simulink model "pvinverter_det"  (R2014a)
settings: Solver=ode23tb  StartTime=0.0  StopTime=0.2  FixedStep=Ts  MaxStep=1e-3  RelTol=1e-4
PreLoadFcn:
  | PVArrayIsc = 5;
  | PVArrayVoc = 21.6;
  | PVArrayRs = 0.036;
  | Tcircuit = 27.15;
  | Toffset = -2;
  | TIPH1 = 0.001;
  | TXIS1 = 3;
  | TRS1 = 0;
  | Ts = 1e-6;
  | load('InvBusObject');
  | load('PVBusObject');
InitFcn:
  | Ts = 1e-6;
StartFcn:
  | tic;
StopFcn:
  | toc;
undefined symbols (not defined in the file or in its folder): sigbuilder_block
libraries: powerlib x13, powerlib_meascontrol x2
settings Model: Creator=cosorio  LastModifiedBy=cosorio
settings DataIOCC: LimitDataPoints=off  SignalLoggingSaveFormat=ModelDataLogs  SaveOutput=off  SignalLogging=off  SaveTime=off
settings OptimizationCC: ExpressionDepthLimit=2147483647
settings DebuggingCC: UnderspecifiedInitializationDetection=Classic  SolverPrmCheckMsg=none  FcnCallInpInsideContextMsg=UseLocalSettings  StateNameClashWarn=warning
settings GRTTargetCC: CombineOutputUpdateFcns=off  GRTInterface=on

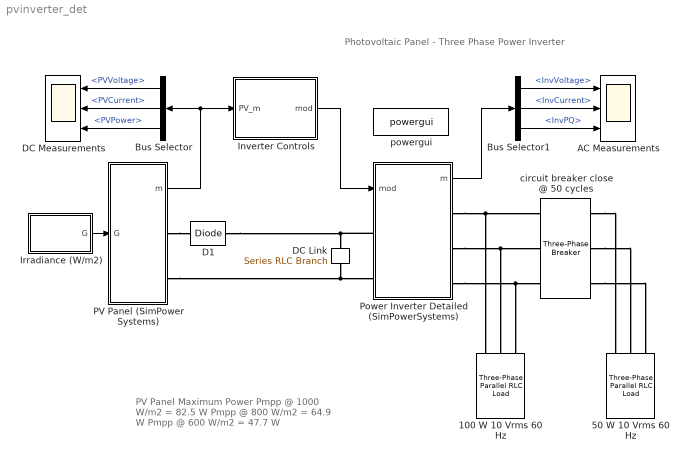
== system pvinverter_det ==
  note: Photovoltaic Panel - Three Phase Power Inverter
  note: PV Panel Maximum Power
      | Pmpp @ 1000 W/m2 = 82.5 W
      | Pmpp @ 800 W/m2 = 64.9 W
      | Pmpp @ 600 W/m2 = 47.7 W
  100 W 10 Vrms 60 Hz : powerlib/Elements/Three-Phase Parallel RLC Load  LConnTagsString=A|B|C  Configuration=Y (grounded)  NominalVoltage=10  NominalFrequency=60  ActivePower=100  InductivePower=0  CapacitivePower=0  Measurements=None  LoadType=constant Z
  50 W 10 Vrms 60 Hz : powerlib/Elements/Three-Phase Parallel RLC Load  LConnTagsString=A|B|C  Configuration=Y (grounded)  NominalVoltage=10  NominalFrequency=60  ActivePower=50  InductivePower=0  CapacitivePower=0  Measurements=None  LoadType=constant Z
  AC Measurements : Scope  NumInputPorts=3
      settings: YMin=-10~-10~0  YMax=10~10~100  SaveName=InverterData
  Bus Selector : BusSelector  OutputSignals=PVVoltage,PVCurrent,PVPower
  Bus Selector1 : BusSelector  OutputSignals=InvVoltage,InvCurrent,InvPQ
  D1 : powerlib/Power Electronics/Diode  Ron=0.001  Lon=0  Vf=0.8  IC=0  UseSnubber=off  Rs=500  Cs=250e-9  Measurements=off
  DC Link : powerlib/Elements/Series RLC Branch  LConnTagsString=__new0  RConnTagsString=__new0  BranchType=C  Resistance=1  Inductance=1e-3  SetiL0=off  InitialCurrent=0  Capacitance=480e-6  Setx0=on  InitialVoltage=18  Measurements=None
  DC Measurements : Scope  NumInputPorts=3
      settings: YMin=0~0~0  YMax=25~6~100
  Inverter Controls : Subsystem  TreatAsAtomicUnit=on  SystemSampleTime=1e-4
  Irradiance (W/m2) : Subsystem  Tag=STV Subsys  LoadFcn=sigbuilder_block('load');  StartFcn=sigbuilder_block('start');  StopFcn=sigbuilder_block('stop');  ClipboardFcn=sigbuilder_block('clipboard');  mask(Sigbuilder block){}
      mask help: Sigbuilder GUI
      mask init:
      | if ~strcmp(get_param(bdroot(gcbh),'SimulationStatus'),'stopped') tuvar = sigbuilder_block('maskInit'); end
      settings: CopyFcn=sigbuilder_block('copy');  DeleteFcn=sigbuilder_block('delete');  ModelCloseFcn=sigbuilder_block('modelClose');  PreSaveFcn=sigbuilder_block('preSave');  PauseFcn=sigbuilder_block('pause')  ContinueFcn=sigbuilder_block('continue')  NameChangeFcn=sigbuilder_block('namechange');  OpenFcn=sigbuilder_block('open',[124.138 46.5517 550.552 391.034 ]);  CloseFcn=sigbuilder_block('close');
      mask Display: plot(0,0,100,100,[10,10,40,40,10],[80,20,20,80,80],[40,10],[50,50], [40,27,10],[65,72,56],[40,25,25,10],[28,28,43,43]);
  PV Panel (SimPowerSystems) : Subsystem
  Power Inverter Detailed (SimPowerSystems) : Subsystem
  circuit breaker close @ 50 cycles : powerlib/Elements/Three-Phase Breaker  InitialState=open  SwitchA=on  SwitchB=on  SwitchC=on  SwitchTimes=[50/60]  External=off  BreakerResistance=0.001  SnubberResistance=1e6  SnubberCapacitance=inf  Measurements=None
  powergui : powerlib/powergui  Priority=1  SimulationMode=Discrete  SolverType=Tustin  SampleTime=Ts  frequency=60  SPID=off  DisableSnubberDevices=off  DisableRonSwitches=off  DisableVfSwitches=off  SwTol=0  Interpol=off  DisplayEquations=off  Ts=0  methode=off  frequencyindice=0  Pbase=100e6  ErrMax=1e-4  Iterations=50  UnitsV=kV  UnitsW=MW  FunctionMessages=off  echomessages=off  HookPort=off  EnableUseOfTLC=off  x0status=blocks  RestoreLinks=warning  ResistiveCurrentMeasurement=off  Frange=[0:2:500]  Ylog=off  Xlog=on  ShowGrid=off  save=off  variable=ZData  structure=0  ZoomFFT=on  StartTime=0.0  cycles=1  DisplayStyle=1  fundamental=60  FreqAxis=off  MaxFrequency=1000  frequencyindicesteady=1  RmsSteady=1  display=off
  wires:
  Irradiance (W/m2)/1(G) -> PV Panel (SimPowerSystems)/1(G)
  PV Panel (SimPowerSystems)/1(m) -> Bus Selector/1, Inverter Controls/1(PV_m)
  Bus Selector/3 -> DC Measurements/3  "<PVPower>"
  Bus Selector/1 -> DC Measurements/1  "<PVVoltage>"
  Bus Selector/2 -> DC Measurements/2  "<PVCurrent>"
  Power Inverter Detailed (SimPowerSystems)/1(m) -> Bus Selector1/1
  Bus Selector1/1 -> AC Measurements/1  "<InvVoltage>"
  Bus Selector1/2 -> AC Measurements/2  "<InvCurrent>"
  Bus Selector1/3 -> AC Measurements/3  "<InvPQ>"
  Inverter Controls/1(mod) -> Power Inverter Detailed (SimPowerSystems)/1(mod)
  connections:
  DC Link/RConn1 -- PV Panel (SimPowerSystems)/RConn2 -- Power Inverter Detailed (SimPowerSystems)/LConn2
  Power Inverter Detailed (SimPowerSystems)/LConn1 -- D1/RConn1 -- DC Link/LConn1
  Power Inverter Detailed (SimPowerSystems)/RConn1 -- 100 W 10 Vrms 60 Hz/LConn1 -- circuit breaker close @ 50 cycles/LConn1
  Power Inverter Detailed (SimPowerSystems)/RConn3 -- 100 W 10 Vrms 60 Hz/LConn3 -- circuit breaker close @ 50 cycles/LConn3
  Power Inverter Detailed (SimPowerSystems)/RConn2 -- 100 W 10 Vrms 60 Hz/LConn2 -- circuit breaker close @ 50 cycles/LConn2
  circuit breaker close @ 50 cycles/RConn1 -- 50 W 10 Vrms 60 Hz/LConn1
  circuit breaker close @ 50 cycles/RConn2 -- 50 W 10 Vrms 60 Hz/LConn2
  circuit breaker close @ 50 cycles/RConn3 -- 50 W 10 Vrms 60 Hz/LConn3
  PV Panel (SimPowerSystems)/RConn1 -- D1/LConn1

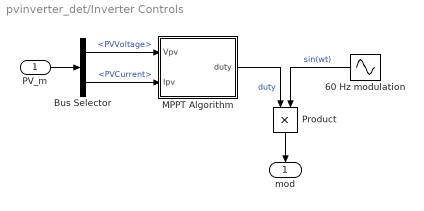
== system pvinverter_det/Inverter Controls ==
  PV_m : Inport
  60 Hz modulation : Sin  Frequency=2*pi*60  Phase=[0, 120*pi/180, -120*pi/180]  SampleTime=1e-4
  Bus Selector : BusSelector  OutputSignals=PVVoltage,PVCurrent
  MPPT Algorithm : Subsystem
  Product : Product  RndMeth=Zero
  mod : Outport
  wires:
  60 Hz modulation/1 -> Product/2  "sin(wt)"
  PV_m/1 -> Bus Selector/1
  Product/1 -> mod/1
  Bus Selector/1 -> MPPT Algorithm/1(Vpv)  "<PVVoltage>"
  Bus Selector/2 -> MPPT Algorithm/2(Ipv)  "<PVCurrent>"
  MPPT Algorithm/1(duty) -> Product/1  "duty"

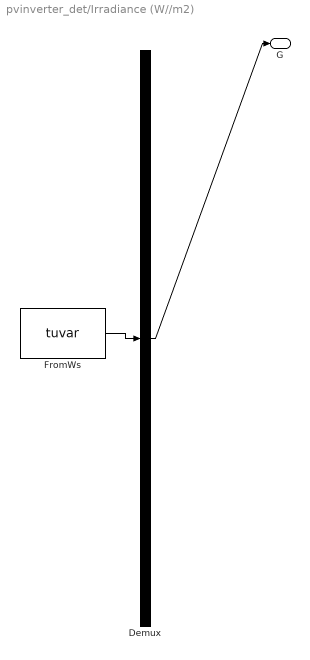
== system pvinverter_det/Irradiance (W//m2) ==
  Demux : Demux  Tag=STV Demux  Outputs=1
  FromWs : FromWorkspace  Tag=STV FromWs  VariableName=tuvar  SampleTime=Ts
      SigBuilderData=|
      | common.afterFinalStr = 'Extrapolate'
      | common.sampleTime = 'Ts'
      | dataSet(1).timeRange = [0 1]
      | dataSet(1).name = 'Constant Irradiance'
      | dataSet(2).timeRange = [0 1]
      | dataSet(2).name = 'Step Irradiance'
      | dataSet(3).timeRange = [0 1]
      | dataSet(3).name = 'Trapezoidal Irradiance'
      | sbobj.Groups(1).Name = 'Constant Irradiance'
      | sbobj.Groups(1).Signals.Name = 'G'
      | sbobj.Groups(1).Signals.XData = [0 1]
      | sbobj.Groups(1).Signals.YData = [800 800]
      | sbobj.Groups(1).TimeRange = [0 1]
      | sbobj.Groups(2).Name = 'Step Irradiance'
      | sbobj.Groups(2).Signals.Name = 'G'
      | sbobj.Groups(2).Signals.XData = [0 0.5 0.5 1]
      | sbobj.Groups(2).Signals.YData = [600 600 1000 1000]
      | sbobj.Groups(2).TimeRange = [0 1]
      | sbobj.Groups(3).Name = 'Trapezoidal Irradiance'
      | sbobj.Groups(3).Signals.Name = 'G'
      | sbobj.Groups(3).Signals.XData = [0 0.2 0.3 0.5 0.7 0.9 1]
      | sbobj.Groups(3).Signals.YData = [800 800 600 600 1000 1000 800]
      | sbobj.Groups(3).TimeRange = [0 1]
  G : Outport  Tag=STV Outport
  wires:
  Demux/1 -> G/1
  FromWs/1 -> Demux/1

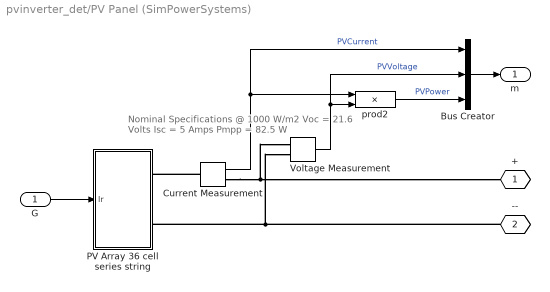
== system pvinverter_det/PV Panel (SimPowerSystems) ==
  note: Nominal Specifications @ 1000 W/m2
      | Voc = 21.6 Volts
      | Isc = 5 Amps
      | Pmpp = 82.5 W
  G : Inport
  Bus Creator : BusCreator  Inputs=3
  Current Measurement : powerlib/Measurements/Current Measurement  PhasorSimulation=off  OutputType=Complex  PSBequivalent=0
  PV Array 36 cell series string : Subsystem  mask(Solar Cell){Isc=5, Voc=0.6*36, Ir0=1000, N=1.5*36, Rs=0.001*36, Rp=1000*36, tau=Ts}
      mask prompts: Isc "Short-circuit current, Isc (A):"; Voc "Open-circuit voltage, Voc (V):"; Ir0 "Irradiance used for measurements, Ir0 (W/m2):"; N "Quality factor, N:"; Rs "Series resistance, Rs (ohms):"; Rp "Parallel resistance, Rp (ohms):"; tau "Time constant (sec):"
      mask help:
      | Simulink implementation of an idividual solar cell. The cell is modelled as a parallel combination of a current source, an exponential diode and an internal resistance Rp, connected in series with a resistance Rs.
      | The cell output current is given by:
      |
      | Ipv = Iph - Is * (exp((V + I*Rs)/(N*Vt)) - 1) - (V + I*Rs)/Rp
      |
      | Where Iph is the solar generated current, Is is the diode saturation current, Vt is the thermal voltage, N is the diode quality factor (emission coefficient).
      |
      | A first order transfer function is used to break the algebraic loop. The time constant of this transfer function should be adjusted such that it will not significantly affect your model dynamics.
      mask init:
      | %% Cell thermal voltage calculation
      | T = 25 + 273;   % Device operating temperature (oC)
      | k = 1.3806e-23; % Boltzman constant (J/oK)
      | q = 1.602e-19;  % Elementary charge on an electron (oC)
      | Vt = k*T/q;     % Thermal voltage
      | 
      | %% Diode saturation current calculation
      | Is = Isc/(exp(Voc/(N*Vt))-1);
  Voltage Measurement : powerlib/Measurements/Voltage Measurement  PhasorSimulation=off  OutputType=Complex  PSBequivalent=0
  prod2 : Product  Inputs=**
  + : PMIOPort  Tag=PMCPort  Port=1  Side=Right
  -- : PMIOPort  Tag=PMCPort  Port=2  Side=Right
  m : Outport
  wires:
  prod2/1 -> Bus Creator/3  "PVPower"
  G/1 -> PV Array 36 cell series string/1(Ir)
  Bus Creator/1 -> m/1
  Voltage Measurement/1 -> prod2/2, Bus Creator/2  "PVVoltage"
  Current Measurement/1 -> prod2/1, Bus Creator/1  "PVCurrent"
  connections:
  --/RConn1 -- PV Array 36 cell series string/RConn2 -- Voltage Measurement/LConn2
  Current Measurement/RConn1 -- +/RConn1 -- Voltage Measurement/LConn1
  Current Measurement/LConn1 -- PV Array 36 cell series string/RConn1

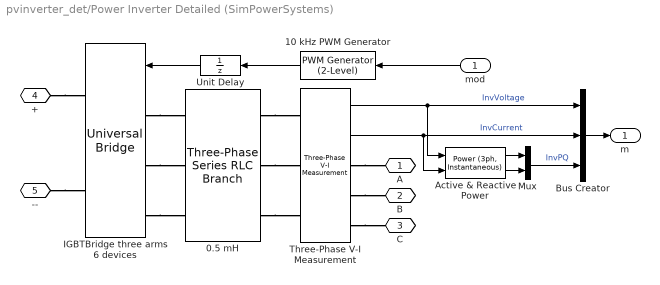
== system pvinverter_det/Power Inverter Detailed (SimPowerSystems) ==
  mod : Inport
  0.5 mH : powerlib/Elements/Three-Phase Series RLC Branch  LConnTagsString=A|B|C  RConnTagsString=A|B|C  BranchType=L  Resistance=1.0  Inductance=500e-6  Capacitance=1.0  Measurements=None
  10 kHz PWM Generator : powerlib_meascontrol/Pulse & Signal Generators/PWM Generator (2-Level)  ModulatorType=Three-phase bridge (6 pulses)  ModulatorMode=Unsynchronized  nF=27  Fc=1e4  ModulatingSignals=off  m=0.8  Freq=60  Phase=0  Ts=Ts
  Active & Reactive Power : powerlib_meascontrol/Measurements/Power (3ph, Instantaneous)
  Bus Creator : BusCreator  Inputs=3
  IGBTBridge three arms 6 devices : powerlib/Power Electronics/Universal Bridge  Arms=3  SnubberResistance=1e5  SnubberCapacitance=inf  Device=IGBT / Diodes  Ron=1e-3  Lon=0  ForwardVoltages="[  0  0  ]"  ForwardVoltage=0  GTOparameters=[ 10e-6 , 20e-6 ]  IGBTparameters=[ 1e-6 , 2e-6 ]  Measurements=None  Measurements_2=None  converterType=Rectifier
  Mux : Mux  Inputs=2
  Three-Phase V-I Measurement : powerlib/Measurements/Three-Phase V-I Measurement  VoltageMeasurement=phase-to-ground  SetLabelV=off  LabelV=Vabc  Vpu=off  VpuLL=off  CurrentMeasurement=yes  SetLabelI=off  LabelI=Iabc  Ipu=off  Pbase=100e6  Vbase=500e3  OutputType=Complex  PhasorSimulation=off  PSBequivalent=0
  Unit Delay : UnitDelay  SampleTime=Ts
  A : PMIOPort  Port=1  Side=Right
  B : PMIOPort  Port=2  Side=Right
  C : PMIOPort  Port=3  Side=Right
  + : PMIOPort  Port=4  Side=Left
  -- : PMIOPort  Port=5  Side=Left
  m : Outport
  wires:
  Three-Phase V-I Measurement/1 -> Bus Creator/1, Active & Reactive Power/1  "InvVoltage"
  Mux/1 -> Bus Creator/3  "InvPQ"
  Three-Phase V-I Measurement/2 -> Bus Creator/2, Active & Reactive Power/2  "InvCurrent"
  Bus Creator/1 -> m/1
  mod/1 -> 10 kHz PWM Generator/1
  Unit Delay/1 -> IGBTBridge three arms 6 devices/1
  Active & Reactive Power/2 -> Mux/2
  Active & Reactive Power/1 -> Mux/1
  10 kHz PWM Generator/1 -> Unit Delay/1
  connections:
  IGBTBridge three arms 6 devices/LConn1 -- 0.5 mH/LConn1
  IGBTBridge three arms 6 devices/LConn2 -- 0.5 mH/LConn2
  IGBTBridge three arms 6 devices/LConn3 -- 0.5 mH/LConn3
  0.5 mH/RConn1 -- Three-Phase V-I Measurement/LConn1
  0.5 mH/RConn2 -- Three-Phase V-I Measurement/LConn2
  0.5 mH/RConn3 -- Three-Phase V-I Measurement/LConn3
  Three-Phase V-I Measurement/RConn1 -- A/RConn1
  Three-Phase V-I Measurement/RConn2 -- B/RConn1
  Three-Phase V-I Measurement/RConn3 -- C/RConn1
  +/RConn1 -- IGBTBridge three arms 6 devices/RConn1
  --/RConn1 -- IGBTBridge three arms 6 devices/RConn2

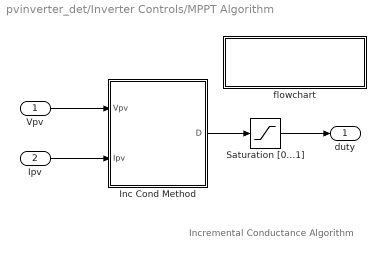
== system pvinverter_det/Inverter Controls/MPPT Algorithm ==
  note: Incremental Conductance Algorithm
  Vpv : Inport  OutDataTypeStr=double  PortDimensions=1  SampleTime=[0.0001,0]
  Ipv : Inport  Port=2  OutDataTypeStr=double  PortDimensions=1  SampleTime=[0.0001,0]
  Inc Cond Method : Stateflow chart  TreatAsAtomicUnit=on
  Saturation [0...1] : Saturate  UpperLimit=1  LowerLimit=0
  flowchart : Subsystem
      settings: OpenFcn=winopen('INC.jpg');
      mask Display: disp('Algorithm\nFlowchart')
  duty : Outport  OutDataTypeStr=double  PortDimensions=1  SampleTime=[0.0001,0]
  wires:
  Inc Cond Method/1(D) -> Saturation [0...1]/1
  Vpv/1 -> Inc Cond Method/1(Vpv)
  Ipv/1 -> Inc Cond Method/2(Ipv)
  Saturation [0...1]/1 -> duty/1

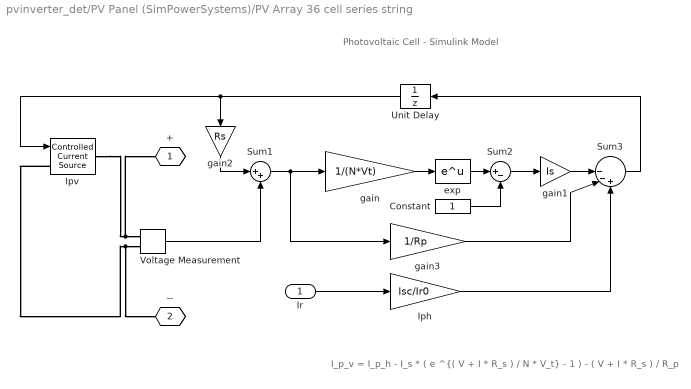
== system pvinverter_det/PV Panel (SimPowerSystems)/PV Array 36 cell series string ==
  note: I_p_v = I_p_h - I_s * ( e ^{( V + I * R_s ) / N * V_t} - 1 ) - ( V + I * R_s ) / R_p
  note: Photovoltaic Cell - Simulink Model
  Ir : Inport
  Constant : Constant
  Iph : Gain  Gain=Isc/Ir0
  Ipv : powerlib/Electrical Sources/Controlled Current Source  Initialize=on  Source_Type=DC  Amplitude=0  Phase=0  Frequency=0  Measurements=None
  Sum1 : Sum  Inputs=|++
  Sum2 : Sum  Inputs=|+-
  Sum3 : Sum  Inputs=||--+
  Unit Delay : UnitDelay  InitialCondition=4.65  SampleTime=tau
  Voltage Measurement : powerlib/Measurements/Voltage Measurement  PhasorSimulation=off  OutputType=Complex  PSBequivalent=0
  exp : Math  SaturateOnIntegerOverflow=on
  gain : Gain  Gain=1/(N*Vt)
  gain1 : Gain  Gain=Is
  gain2 : Gain  Gain=Rs
  gain3 : Gain  Gain=1/Rp
  + : PMIOPort  Tag=PMCPort  Port=1  Side=Right
  -- : PMIOPort  Tag=PMCPort  Port=2  Side=Right
  wires:
  Sum2/1 -> gain1/1
  Constant/1 -> Sum2/2
  exp/1 -> Sum2/1
  Sum1/1 -> gain/1, gain3/1
  gain/1 -> exp/1
  Sum3/1 -> Unit Delay/1
  Voltage Measurement/1 -> Sum1/2
  Ir/1 -> Iph/1
  Unit Delay/1 -> gain2/1, Ipv/1
  gain2/1 -> Sum1/1
  gain1/1 -> Sum3/1
  gain3/1 -> Sum3/2
  Iph/1 -> Sum3/3
  connections:
  Voltage Measurement/LConn1 -- +/RConn1 -- Ipv/RConn1
  Voltage Measurement/LConn2 -- --/RConn1 -- Ipv/LConn1

== system pvinverter_det/Inverter Controls/MPPT Algorithm/flowchart ==

== stateflow chart pvinverter_det/Inverter Controls/MPPT Algorithm/Inc Cond Method ==
  settings: updateMethod=DISCRETE  sampleTime=1e-4
  state SAMPLEandCALCULATE
    entry:
    deltaV = Vpv - Vprev;
    deltaI = Ipv - Iprev;
    d = D;
  state INCREMENT_DUTY
    entry:
    d = d + deltad;
  state DECREMENT_DUTY
    entry:
    d = d - deltad;
  state RETURN
    entry:
    Vprev = Vpv; Iprev = Ipv;
    D = d;
  RETURN -> SAMPLEandCALCULATE
  (default) -> SAMPLEandCALCULATE
  SAMPLEandCALCULATE -> (junction 14) [order 1] : [deltaV > Vtol || deltaV < -Vtol]
  SAMPLEandCALCULATE -> (junction 15) [order 2]
  (junction 15) -> RETURN [order 3]
  (junction 15) -> INCREMENT_DUTY [order 1] : [deltaI < -Itol]
  (junction 14) -> RETURN [order 3]
  (junction 14) -> DECREMENT_DUTY [order 1] : [deltaI/deltaV > -Ipv/Vpv]
  (junction 14) -> INCREMENT_DUTY [order 2] : [deltaI/deltaV < -Ipv/Vpv]
  (junction 15) -> DECREMENT_DUTY [order 2] : [deltaI > Itol]
  INCREMENT_DUTY -> RETURN
  DECREMENT_DUTY -> RETURN
  data: Vpv input; Ipv input; D output double =0.8; Vprev local double =0; Iprev local double =0; Itol constant double =0.001; Vtol constant double =0.001; deltad constant double =0.0025; deltaV local double =0; deltaI local double =0; d local double =0
